simulink model "pmsm_drive_2_Ref_Design_02ms"  (R2013b)
settings: Solver=ode45  StartTime=0.0  StopTime=0.2  MaxStep=0.000001  MinStep=0.0000001  RelTol=1e-3
libraries: powerlib x5, simulink x3
settings Model: Creator=User  LastModifiedBy=User
settings SolverCC: ZeroCrossControl=DisableAll
settings ConfigurationSet: Description=SimMechanics 2G

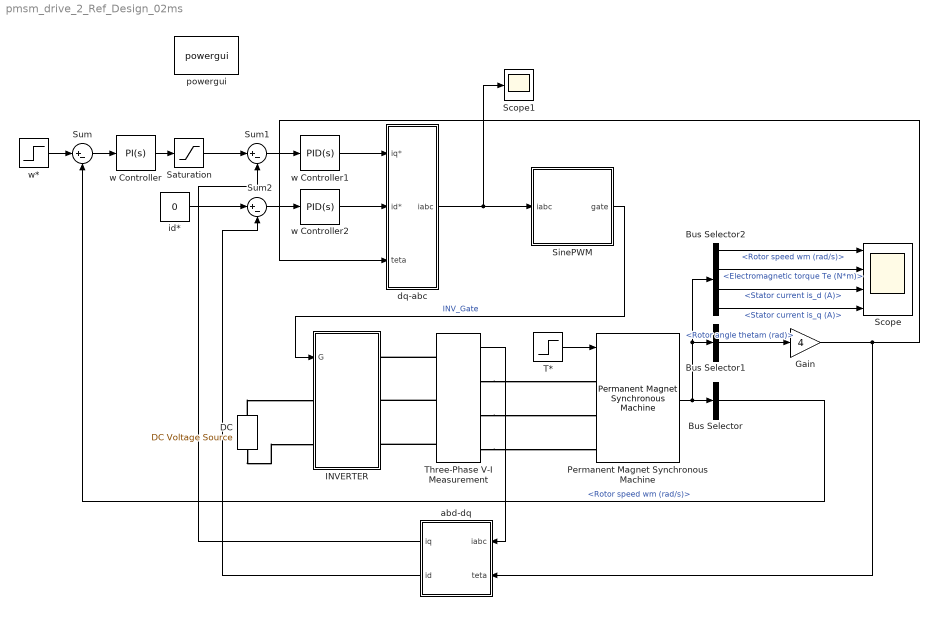
== system pmsm_drive_2_Ref_Design_02ms ==
  Bus Selector : BusSelector  OutputSignals=Rotor speed wm (rad/s)
  Bus Selector1 : BusSelector  OutputSignals=Rotor angle thetam (rad)
  Bus Selector2 : BusSelector  OutputSignals=Rotor speed wm (rad/s),Electromagnetic torque Te (N*m),Stator current is_d (A),Stator current is_q (A)
  DC : powerlib/Electrical Sources/DC Voltage Source  Amplitude=400  Measurements=None
  Gain : Gain  Gain=4
  INVERTER : Subsystem
  Permanent Magnet Synchronous Machine : powerlib/Machines/Permanent Magnet Synchronous Machine  NbPhases=3  FluxDistribution=Sinusoidal  RotorType=Salient-pole  MechanicalLoad=Torque Tm  PresetModel=No  ShowDetailedParameters=on  Resistance=0.61  Inductance=8.5e-3  dqInductances=[9.1e-3,11.5e-3]  La=0.000835  MachineConstant=Flux linkage established by magnets (V.s)  Flux=0.175  VoltageCst=126.966  TorqueCst=1.05  Flat=120  Mechanical=[0.0027 0.0004924 4 0.01]  PolePairs=4  InitialConditions=[0,0, 0,0]  InitialConditions5ph=[0 0 0 0 0 0]  TsPowergui=0  TsBlock=-1  RefAngle=90 degrees behind phase A axis (modified Park)
  Saturation : Saturate  UpperLimit=15  LowerLimit=-15
  Scope : Scope  NumInputPorts=4
      settings: YMin=101.702~-10.01~-0.15~-9.52  YMax=101.709~-9.88~-0.03~-9.4
  Scope1 : Scope
      settings: YMin=-2000  YMax=2000
  SinePWM : Subsystem
  Sum : Sum  Inputs=|+-
  Sum1 : Sum  Inputs=|+-
  Sum2 : Sum  Inputs=|+-
  T* : Step  Time=0.2  Before=-10  After=-10  SampleTime=0
  Three-Phase V-I Measurement : powerlib/Measurements/Three-Phase V-I Measurement  VoltageMeasurement=no  SetLabelV=off  LabelV=Vabc  Vpu=off  VpuLL=off  CurrentMeasurement=yes  SetLabelI=off  LabelI=Iabc  Ipu=off  Pbase=100e6  Vbase=500e3  OutputType=Complex  PhasorSimulation=off  PSBequivalent=0
  abd-dq : Subsystem
  dq-abc : Subsystem
  id* : Constant  Value=0
  powergui : powerlib/powergui  Priority=1  SimulationMode=Continuous  SolverType=Tustin  SampleTime=50e-6  frequency=60  SPID=off  DisableSnubberDevices=off  DisableRonSwitches=off  DisableVfSwitches=off  SwTol=0  Interpol=off  DisplayEquations=off  frequencyindice=0  Pbase=100e6  ErrMax=1e-4  Iterations=50  UnitsV=kV  UnitsW=MW  FunctionMessages=off  echomessages=off  HookPort=off  EnableUseOfTLC=off  x0status=blocks  RestoreLinks=warning  ResistiveCurrentMeasurement=off  Frange=[0:2:500]  Ylog=off  Xlog=on  ShowGrid=off  save=off  variable=ZData  structure=ScopeData1  ZoomFFT=on  StartTime=0.02  cycles=10  DisplayStyle=1  fundamental=65  FreqAxis=on  MaxFrequency=1000  frequencyindicesteady=1  RmsSteady=1  display=off  Ts=0  methode=off
  w Controller : simulink/Continuous/PID Controller  Controller=PI  TimeDomain=Continuous-time  SampleTime=1  IntegratorMethod=Forward Euler  FilterMethod=Forward Euler  Form=Parallel  P=6  I=2.5  D=0  N=100  InitialConditionSource=internal  InitialConditionForIntegrator=0  InitialConditionForFilter=0  ExternalReset=none  LimitOutput=off  UpperSaturationLimit=inf  LowerSaturationLimit=-inf  LinearizeAsGain=on  AntiWindupMode=none  Kb=1  TrackingMode=off  Kt=1  PParamMin=[]  PParamMax=[]  IParamMin=[]  IParamMax=[]  DParamMin=[]  DParamMax=[]  NParamMin=[]  NParamMax=[]  KbParamMin=[]  KbParamMax=[]  KtParamMin=[]  KtParamMax=[]  POutMin=[]  POutMax=[]  IOutMin=[]  IOutMax=[]  DOutMin=[]  DOutMax=[]  NOutMin=[]  NOutMax=[]  KbOutMin=[]  KbOutMax=[]  KtOutMin=[]  KtOutMax=[]  IntegratorOutMin=[]  IntegratorOutMax=[]  FilterOutMin=[]  FilterOutMax=[]  SumOutMin=[]  SumOutMax=[]  SumI1OutMin=[]  SumI1OutMax=[]  SumI2OutMin=[]  SumI2OutMax=[]  SumI3OutMin=[]  SumI3OutMax=[]  SumDOutMin=[]  SumDOutMax=[]  SaturationOutMin=[]  SaturationOutMax=[]  IntegratorContinuousStateAttributes=''  IntegratorStateMustResolveToSignalObject=off  IntegratorRTWStateStorageClass=Auto  FilterContinuousStateAttributes=''  FilterStateMustResolveToSignalObject=off  FilterRTWStateStorageClass=Auto
  w Controller1 : simulink/Continuous/PID Controller  Controller=PID  TimeDomain=Continuous-time  SampleTime=1  IntegratorMethod=Forward Euler  FilterMethod=Forward Euler  Form=Parallel  P=3  I=3  D=5  N=100  InitialConditionSource=internal  InitialConditionForIntegrator=0  InitialConditionForFilter=0  ExternalReset=none  LimitOutput=off  UpperSaturationLimit=inf  LowerSaturationLimit=-inf  LinearizeAsGain=on  AntiWindupMode=none  Kb=1  TrackingMode=off  Kt=1  PParamMin=[]  PParamMax=[]  IParamMin=[]  IParamMax=[]  DParamMin=[]  DParamMax=[]  NParamMin=[]  NParamMax=[]  KbParamMin=[]  KbParamMax=[]  KtParamMin=[]  KtParamMax=[]  POutMin=[]  POutMax=[]  IOutMin=[]  IOutMax=[]  DOutMin=[]  DOutMax=[]  NOutMin=[]  NOutMax=[]  KbOutMin=[]  KbOutMax=[]  KtOutMin=[]  KtOutMax=[]  IntegratorOutMin=[]  IntegratorOutMax=[]  FilterOutMin=[]  FilterOutMax=[]  SumOutMin=[]  SumOutMax=[]  SumI1OutMin=[]  SumI1OutMax=[]  SumI2OutMin=[]  SumI2OutMax=[]  SumI3OutMin=[]  SumI3OutMax=[]  SumDOutMin=[]  SumDOutMax=[]  SaturationOutMin=[]  SaturationOutMax=[]  IntegratorContinuousStateAttributes=''  IntegratorStateMustResolveToSignalObject=off  IntegratorRTWStateStorageClass=Auto  FilterContinuousStateAttributes=''  FilterStateMustResolveToSignalObject=off  FilterRTWStateStorageClass=Auto
  w Controller2 : simulink/Continuous/PID Controller  Controller=PID  TimeDomain=Continuous-time  SampleTime=1  IntegratorMethod=Forward Euler  FilterMethod=Forward Euler  Form=Parallel  P=7  I=2.5  D=5  N=100  InitialConditionSource=internal  InitialConditionForIntegrator=0  InitialConditionForFilter=0  ExternalReset=none  LimitOutput=off  UpperSaturationLimit=inf  LowerSaturationLimit=-inf  LinearizeAsGain=on  AntiWindupMode=none  Kb=1  TrackingMode=off  Kt=1  PParamMin=[]  PParamMax=[]  IParamMin=[]  IParamMax=[]  DParamMin=[]  DParamMax=[]  NParamMin=[]  NParamMax=[]  KbParamMin=[]  KbParamMax=[]  KtParamMin=[]  KtParamMax=[]  POutMin=[]  POutMax=[]  IOutMin=[]  IOutMax=[]  DOutMin=[]  DOutMax=[]  NOutMin=[]  NOutMax=[]  KbOutMin=[]  KbOutMax=[]  KtOutMin=[]  KtOutMax=[]  IntegratorOutMin=[]  IntegratorOutMax=[]  FilterOutMin=[]  FilterOutMax=[]  SumOutMin=[]  SumOutMax=[]  SumI1OutMin=[]  SumI1OutMax=[]  SumI2OutMin=[]  SumI2OutMax=[]  SumI3OutMin=[]  SumI3OutMax=[]  SumDOutMin=[]  SumDOutMax=[]  SaturationOutMin=[]  SaturationOutMax=[]  IntegratorContinuousStateAttributes=''  IntegratorStateMustResolveToSignalObject=off  IntegratorRTWStateStorageClass=Auto  FilterContinuousStateAttributes=''  FilterStateMustResolveToSignalObject=off  FilterRTWStateStorageClass=Auto
  w* : Step  Time=0.2  Before=100  After=100  SampleTime=0
  wires:
  Sum/1 -> w Controller/1
  w*/1 -> Sum/1
  Permanent Magnet Synchronous Machine/1 -> Bus Selector/1, Bus Selector1/1, Bus Selector2/1
  Bus Selector/1 -> Sum/2  "<Rotor speed wm (rad/s)>"
  Bus Selector1/1 -> Gain/1  "<Rotor angle thetam (rad)>"
  Bus Selector2/1 -> Scope/1  "<Rotor speed wm (rad/s)>"
  Bus Selector2/2 -> Scope/2  "<Electromagnetic torque Te (N*m)>"
  Bus Selector2/3 -> Scope/3  "<Stator current is_d (A)>"
  Bus Selector2/4 -> Scope/4  "<Stator current is_q (A)>"
  T*/1 -> Permanent Magnet Synchronous Machine/1
  w Controller/1 -> Saturation/1
  Saturation/1 -> Sum1/1
  Sum1/1 -> w Controller1/1
  w Controller1/1 -> dq-abc/1(iq*)
  id*/1 -> Sum2/1
  Sum2/1 -> w Controller2/1
  w Controller2/1 -> dq-abc/2(id*)
  Gain/1 -> abd-dq/2(teta), dq-abc/3(teta)
  SinePWM/1(gate) -> INVERTER/1(G)  "INV_Gate"
  Three-Phase V-I Measurement/1 -> abd-dq/1(iabc)
  abd-dq/1(iq) -> Sum1/2
  abd-dq/2(id) -> Sum2/2
  dq-abc/1(iabc) -> Scope1/1, SinePWM/1(iabc)
  connections:
  Three-Phase V-I Measurement/LConn1 -- INVERTER/RConn1
  Three-Phase V-I Measurement/LConn2 -- INVERTER/RConn2
  Three-Phase V-I Measurement/LConn3 -- INVERTER/RConn3
  Three-Phase V-I Measurement/RConn1 -- Permanent Magnet Synchronous Machine/LConn1
  Three-Phase V-I Measurement/RConn2 -- Permanent Magnet Synchronous Machine/LConn2
  Three-Phase V-I Measurement/RConn3 -- Permanent Magnet Synchronous Machine/LConn3
  DC/RConn1 -- INVERTER/LConn1
  DC/LConn1 -- INVERTER/LConn2

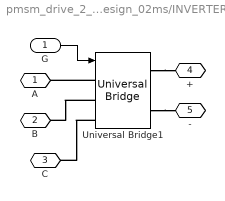
== system pmsm_drive_2_Ref_Design_02ms/INVERTER ==
  G : Inport
  Universal Bridge1 : powerlib/Power Electronics/Universal Bridge  Arms=3  SnubberResistance=1e5  SnubberCapacitance=inf  Device=IGBT / Diodes  Ron=1e-3  Lon=0  ForwardVoltages="[  0  0  ]"  ForwardVoltage=0  GTOparameters=[ 10e-6 , 20e-6 ]  IGBTparameters=[ 1e-6 , 2e-6 ]  Measurements=None  Measurements_2=None  converterType=Rectifier
  A : PMIOPort  Port=1  Side=Right
  B : PMIOPort  Port=2  Side=Right
  C : PMIOPort  Port=3  Side=Right
  + : PMIOPort  Port=4  Side=Left
  - : PMIOPort  Port=5  Side=Left
  wires:
  G/1 -> Universal Bridge1/1
  connections:
  Universal Bridge1/RConn2 -- -/RConn1
  Universal Bridge1/RConn1 -- +/RConn1
  Universal Bridge1/LConn3 -- C/RConn1
  Universal Bridge1/LConn2 -- B/RConn1
  Universal Bridge1/LConn1 -- A/RConn1

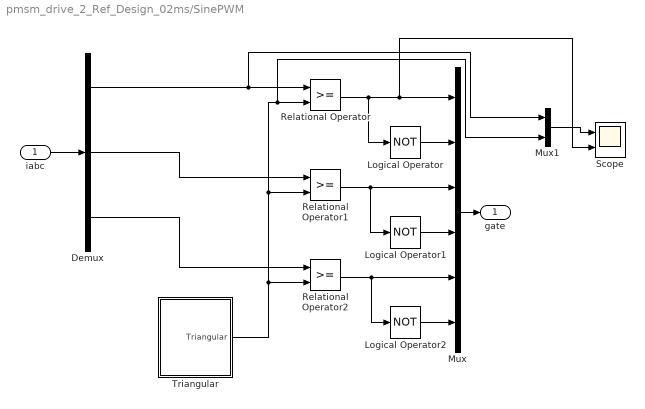
== system pmsm_drive_2_Ref_Design_02ms/SinePWM ==
  iabc : Inport
  Demux : Demux  Outputs=3
  Logical Operator : Logic  Operator=NOT  AllPortsSameDT=off  OutDataTypeStr=boolean
  Logical Operator1 : Logic  Operator=NOT  AllPortsSameDT=off  OutDataTypeStr=boolean
  Logical Operator2 : Logic  Operator=NOT  AllPortsSameDT=off  OutDataTypeStr=boolean
  Mux : Mux  Inputs=6
  Mux1 : Mux  Inputs=2
  Relational Operator : RelationalOperator  OutDataTypeStr=boolean
  Relational Operator1 : RelationalOperator  OutDataTypeStr=boolean
  Relational Operator2 : RelationalOperator  OutDataTypeStr=boolean
  Scope : Scope  NumInputPorts=2
      settings: YMin=-450~-0.5  YMax=450~1.5  SaveName=ScopeData2
  Triangular : Subsystem
  gate : Outport
  wires:
  Demux/1 -> Mux1/1, Relational Operator/1
  Demux/3 -> Relational Operator2/1
  Relational Operator1/1 -> Logical Operator1/1, Mux/3
  Mux/1 -> gate/1
  Logical Operator1/1 -> Mux/4
  Relational Operator2/1 -> Logical Operator2/1, Mux/5
  iabc/1 -> Demux/1
  Demux/2 -> Relational Operator1/1
  Logical Operator/1 -> Mux/2
  Logical Operator2/1 -> Mux/6
  Relational Operator/1 -> Logical Operator/1, Scope/2, Mux/1
  Triangular/1(Triangular) -> Mux1/2, Relational Operator/2, Relational Operator1/2, Relational Operator2/2
  Mux1/1 -> Scope/1

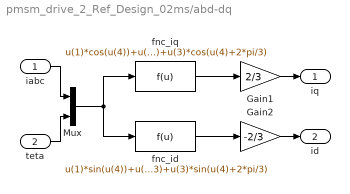
== system pmsm_drive_2_Ref_Design_02ms/abd-dq ==
  iabc : Inport
  teta : Inport  Port=2
  Gain1 : Gain  Gain=2/3
  Gain2 : Gain  Gain=-2/3
  Mux : Mux  Inputs=2
  fnc_id : Fcn  Expr=u(1)*sin(u(4))+u(2)*sin(u(4)-2*pi/3)+u(3)*sin(u(4)+2*pi/3)
  fnc_iq : Fcn  Expr=u(1)*cos(u(4))+u(2)*cos(u(4)-2*pi/3)+u(3)*cos(u(4)+2*pi/3)
  iq : Outport
  id : Outport  Port=2
  wires:
  fnc_id/1 -> Gain2/1
  Gain1/1 -> iq/1
  teta/1 -> Mux/2
  iabc/1 -> Mux/1
  Mux/1 -> fnc_iq/1, fnc_id/1
  Gain2/1 -> id/1
  fnc_iq/1 -> Gain1/1

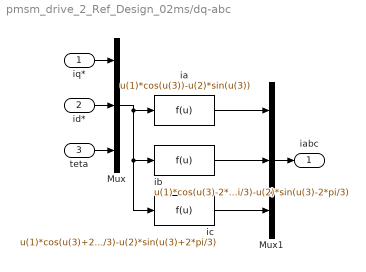
== system pmsm_drive_2_Ref_Design_02ms/dq-abc ==
  iq* : Inport
  id* : Inport  Port=2
  teta : Inport  Port=3
  Mux : Mux  Inputs=3
  Mux1 : Mux  Inputs=3
  ia : Fcn  Expr=u(1)*cos(u(3))-u(2)*sin(u(3))
  ib : Fcn  Expr=u(1)*cos(u(3)-2*pi/3)-u(2)*sin(u(3)-2*pi/3)
  ic : Fcn  Expr=u(1)*cos(u(3)+2*pi/3)-u(2)*sin(u(3)+2*pi/3)
  iabc : Outport
  wires:
  id*/1 -> Mux/2
  ia/1 -> Mux1/1
  ib/1 -> Mux1/2
  teta/1 -> Mux/3
  Mux1/1 -> iabc/1
  ic/1 -> Mux1/3
  iq*/1 -> Mux/1
  Mux/1 -> ic/1, ib/1, ia/1

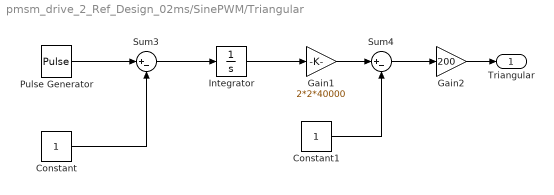
== system pmsm_drive_2_Ref_Design_02ms/SinePWM/Triangular ==
  Constant : Constant
  Constant1 : Constant
  Gain1 : Gain  Gain=2*2*40000
  Gain2 : Gain  Gain=200
  Integrator : Integrator
  Pulse Generator : DiscretePulseGenerator  PulseType=Time based  Amplitude=2  Period=1/40000  PulseWidth=50
  Sum3 : Sum  Inputs=|+-
  Sum4 : Sum  Inputs=|+-
  Triangular : Outport
  wires:
  Pulse Generator/1 -> Sum3/1
  Constant1/1 -> Sum4/2
  Constant/1 -> Sum3/2
  Sum3/1 -> Integrator/1
  Integrator/1 -> Gain1/1
  Gain1/1 -> Sum4/1
  Gain2/1 -> Triangular/1
  Sum4/1 -> Gain2/1
